simulink model "z9"  (R2021a)
settings: Solver=VariableStepAuto  StartTime=0.0  StopTime=50.0  RelTol=1e-3
values from neighbouring files (symbols this model uses):
  T = 0.5    [z3_czas_probkowania_T.m]    (also in z9_czas_probkowania_T_wartosc_ud.m = 1)
  ud = [-1:0.1:1]    [z11_transmitacja_wykres.m]    (also in z6_zlinearyzowana_charakterystyka_statyczna.m = -1; z9_czas_probkowania_T_wartosc_ud.m = 0.5)
settings Model: Creator=48604  LastModifiedBy=48604

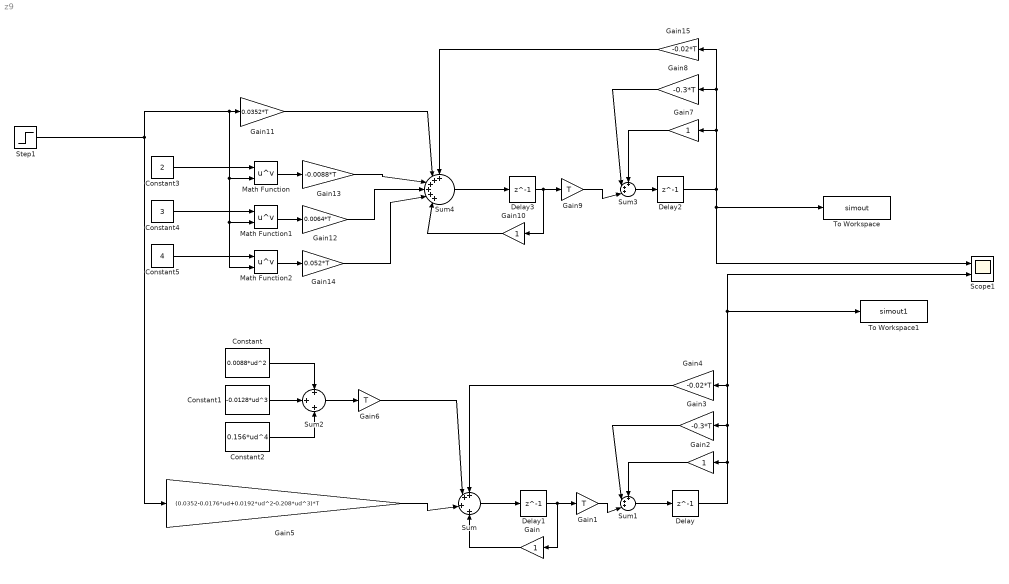
== system z9 ==
  Constant : Constant  Value=0.0088*ud^2
  Constant1 : Constant  Value=-0.0128*ud^3
  Constant2 : Constant  Value=0.156*ud^4
  Constant3 : Constant  Value=2
  Constant4 : Constant  Value=3
  Constant5 : Constant  Value=4
  Delay{,1..3} (4 alike) : Delay  DelayLength=1  InitialCondition=0  SampleTime=1
  Gain{,2,7,10} (4 alike) : Gain
  Gain1 : Gain  Gain=T
  Gain11 : Gain  Gain=0.0352*T
  Gain12 : Gain  Gain=0.0064*T
  Gain13 : Gain  Gain=-0.0088*T
  Gain14 : Gain  Gain=0.052*T
  Gain15 : Gain  Gain=-0.02*T
  Gain3 : Gain  Gain=-0.3*T
  Gain4 : Gain  Gain=-0.02*T
  Gain5 : Gain  Gain=(0.0352-0.0176*ud+0.0192*ud^2-0.208*ud^3)*T
  Gain6 : Gain  Gain=T
  Gain8 : Gain  Gain=-0.3*T
  Gain9 : Gain  Gain=T
  Math Function : Math  Operator=pow  SaturateOnIntegerOverflow=on
  Math Function1 : Math  Operator=pow  SaturateOnIntegerOverflow=on
  Math Function2 : Math  Operator=pow  SaturateOnIntegerOverflow=on
  Scope1 : Scope  NumInputPorts=2
  Step1 : Step  After=0.5  SampleTime=1
  Sum : Sum  Inputs=++|+|+
  Sum1 : Sum  Inputs=+++|
  Sum2 : Sum  Inputs=+|+|+
  Sum3 : Sum  Inputs=+++|
  Sum4 : Sum  Inputs=++++++|
  To Workspace : ToWorkspace  VariableName=simout  SaveFormat=Structure With Time  SampleTime=1
  To Workspace1 : ToWorkspace  VariableName=simout1  SaveFormat=Structure With Time  SampleTime=1
  wires:
  Delay1/1 -> Gain/1, Gain1/1
  Gain1/1 -> Sum1/3
  Delay/1 -> Scope1/2, To Workspace1/1, Gain4/1, Gain3/1, Gain2/1
  Sum1/1 -> Delay/1
  Gain3/1 -> Sum1/2
  Gain2/1 -> Sum1/1
  Sum/1 -> Delay1/1
  Step1/1 -> Gain5/1, Math Function2/2, Math Function1/2, Math Function/2, Gain11/1
  Constant/1 -> Sum2/1
  Constant1/1 -> Sum2/2
  Constant2/1 -> Sum2/3
  Sum2/1 -> Gain6/1
  Gain/1 -> Sum/4
  Gain5/1 -> Sum/3
  Gain6/1 -> Sum/2
  Gain4/1 -> Sum/1
  Gain11/1 -> Sum4/2
  Constant4/1 -> Math Function1/1
  Delay3/1 -> Gain10/1, Gain9/1
  Math Function/1 -> Gain13/1
  Delay2/1 -> Gain8/1, Gain15/1, Gain7/1, To Workspace/1, Scope1/1
  Math Function1/1 -> Gain12/1
  Gain7/1 -> Sum3/1
  Sum3/1 -> Delay2/1
  Gain15/1 -> Sum4/1
  Math Function2/1 -> Gain14/1
  Gain10/1 -> Sum4/6
  Constant3/1 -> Math Function/1
  Gain12/1 -> Sum4/4
  Sum4/1 -> Delay3/1
  Gain9/1 -> Sum3/3
  Constant5/1 -> Math Function2/1
  Gain13/1 -> Sum4/3
  Gain14/1 -> Sum4/5
  Gain8/1 -> Sum3/2
